simulink model "Envloads"  (R2021a)
settings: Solver=VariableStepAuto  StartTime=0.0  StopTime=100  RelTol=1e-3
undefined symbols (not defined in the file): alpha, C_phi, C_psi, C_tetha, Current_dir, Current_vel, Cx, Cy, mu, Umean, wind_dir_mean
libraries: mssSimulink x5, simulink x2
settings Model: Creator=premr  LastModifiedBy=premr

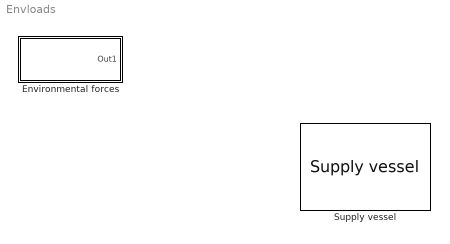
== system Envloads ==
  Environmental forces : Subsystem
  Supply vessel : mssSimulink/Marine craft models/Supply vessel  D=[5.0242e4 0 0; 0 2.7229e5 -4.3933e6; 0 -4.3933e6 4.1894e8]  Minv=inv( [5.3122e6 0 0; 0 8.2831e6 0; 0 0 3.7454e9] )

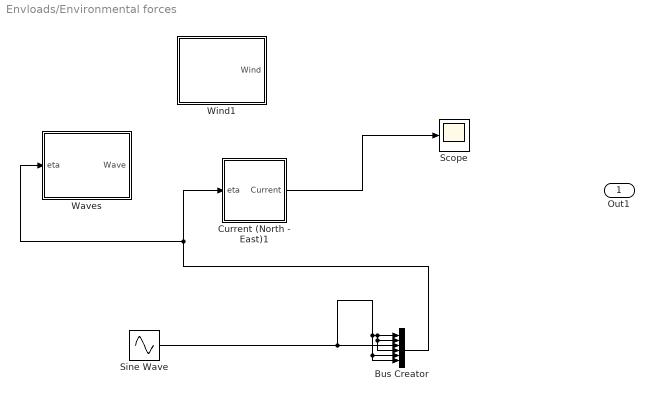
== system Envloads/Environmental forces ==
  Bus Creator : BusCreator  Inputs=6
  Current (North - East)1 : Subsystem
  Scope : Scope
  Sine Wave : Sin  Frequency=1/30  SampleTime=0
  Waves : Subsystem
  Wind1 : Subsystem
  Out1 : Outport
  wires:
  Sine Wave/1 -> Bus Creator/6, Bus Creator/5, Bus Creator/4, Bus Creator/2, Bus Creator/1, Bus Creator/3
  Bus Creator/1 -> Waves/1(eta), Current (North - East)1/1(eta)
  Current (North - East)1/1(Current) -> Scope/1

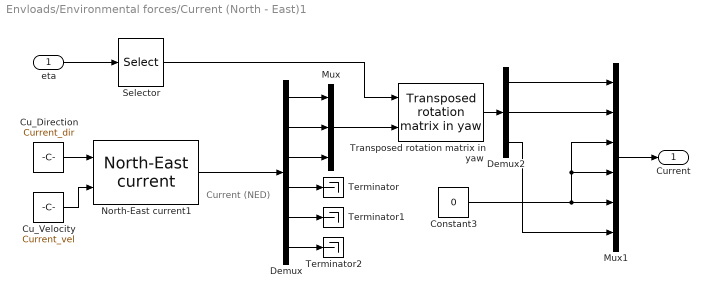
== system Envloads/Environmental forces/Current (North - East)1 ==
  note: Current (NED)
  eta : Inport
  Constant3 : Constant  Value=0
  Cu_Direction : Constant  Value=Current_dir
  Cu_Velocity : Constant  Value=Current_vel
  Demux : Demux  Outputs=6
  Demux2 : Demux  Outputs=3
  Mux : Mux  Inputs=3
  Mux1 : Mux  Inputs=6
  North-East current1 : mssSimulink/Environment/Current/North-East current  SystemSampleTime=-1  VariantActivationTime=update diagram  Latency=0  AutoFrameSizeCalculation=off
  Selector : Selector  InputPortWidth=6  IndexOptions=Index vector (dialog)  Indices=[6]  OutputSizes=1
  Terminator : Terminator
  Terminator1 : Terminator
  Terminator2 : Terminator
  Transposed rotation matrix in yaw : mssSimulink/Modelling/Kinematics/Transposed rotation  matrix in yaw
  Current : Outport  VectorParamsAs1DForOutWhenUnconnected=off
  wires:
  Constant3/1 -> Mux1/5, Mux1/4, Mux1/3
  Demux/6 -> Terminator2/1
  North-East current1/1 -> Demux/1
  Demux2/3 -> Mux1/6
  Demux/4 -> Terminator/1
  Demux/5 -> Terminator1/1
  Selector/1 -> Transposed rotation matrix in yaw/1
  Demux/3 -> Mux/3
  Mux/1 -> Transposed rotation matrix in yaw/2
  Demux/1 -> Mux/1
  Cu_Velocity/1 -> North-East current1/2
  Demux/2 -> Mux/2
  Mux1/1 -> Current/1
  Demux2/2 -> Mux1/2
  Transposed rotation matrix in yaw/1 -> Demux2/1
  eta/1 -> Selector/1
  Cu_Direction/1 -> North-East current1/1
  Demux2/1 -> Mux1/1

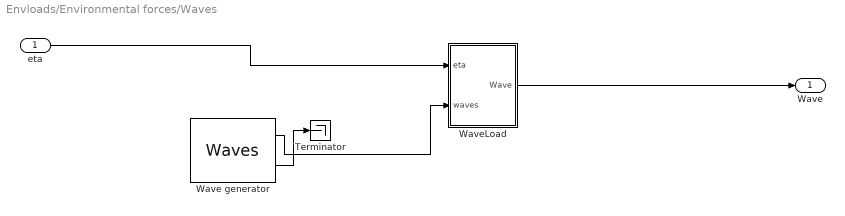
== system Envloads/Environmental forces/Waves ==
  eta : Inport
  Terminator : Terminator
  Wave generator : mssSimulink/Environment/Waves/Waves  spectrum_type=ITTC  disp_flag=on  plot_spectrum=off  plot_realization=off  hs=0.8  omega_peak=0  psi_mean=0  gamma=-1  spread=2  depth=inf  nfreq=20  ndir=10  energylim=0.005  freq_cutoff=3  dir_cutoff=0  rand_seed=123  rand_freq=on  rand_dir=on  Zeta_a=0  Omega=0  Phase=0  Wavenum=0  Psi=0
  WaveLoad : Subsystem  mask{waveforces=on}
      mask prompts: waveforces "Waveforces enabled"
  Wave : Outport  VectorParamsAs1DForOutWhenUnconnected=off
  wires:
  Wave generator/1 -> WaveLoad/2(waves)
  Wave generator/2 -> Terminator/1
  eta/1 -> WaveLoad/1(eta)
  WaveLoad/1(Wave) -> Wave/1

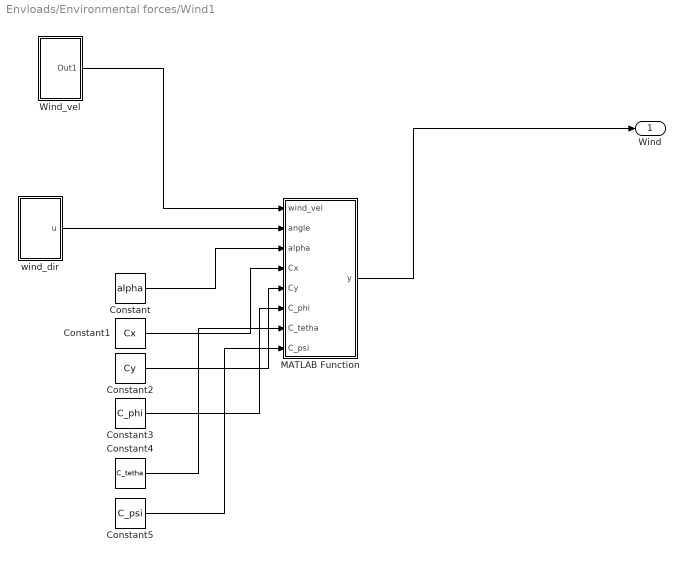
== system Envloads/Environmental forces/Wind1 ==
  Constant : Constant  Value=alpha
  Constant1 : Constant  Value=Cx
  Constant2 : Constant  Value=Cy
  Constant3 : Constant  Value=C_phi
  Constant4 : Constant  Value=C_tetha
  Constant5 : Constant  Value=C_psi
  MATLAB Function : MATLAB Function  TreatAsAtomicUnit=on
  Wind_vel : Subsystem
  wind_dir : Subsystem
  Wind : Outport  VectorParamsAs1DForOutWhenUnconnected=off
  wires:
  wind_dir/1(u) -> MATLAB Function/2(angle)
  Wind_vel/1(Out1) -> MATLAB Function/1(wind_vel)
  MATLAB Function/1(y) -> Wind/1
  Constant/1 -> MATLAB Function/3(alpha)
  Constant1/1 -> MATLAB Function/4(Cx)
  Constant2/1 -> MATLAB Function/5(Cy)
  Constant3/1 -> MATLAB Function/6(C_phi)
  Constant4/1 -> MATLAB Function/7(C_tetha)
  Constant5/1 -> MATLAB Function/8(C_psi)

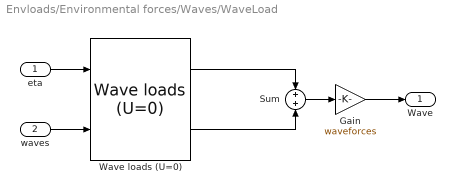
== system Envloads/Environmental forces/Waves/WaveLoad ==
  eta : Inport
  waves : Inport  Port=2
  Gain : Gain  Gain=waveforces
  Sum : Sum
  Wave loads (U=0) : mssSimulink/Hydrodynamics/Wave loads (U=0)  SystemSampleTime=-1  VariantActivationTime=update diagram  Latency=0  AutoFrameSizeCalculation=off
  Wave : Outport  VectorParamsAs1DForOutWhenUnconnected=off
  wires:
  eta/1 -> Wave loads (U=0)/1
  waves/1 -> Wave loads (U=0)/2
  Sum/1 -> Gain/1
  Wave loads (U=0)/1 -> Sum/1
  Wave loads (U=0)/2 -> Sum/2
  Gain/1 -> Wave/1

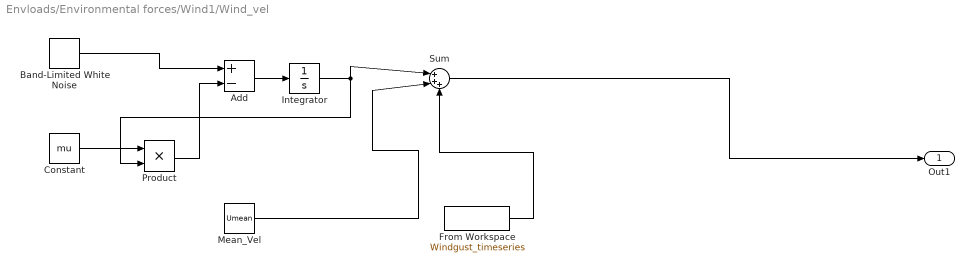
== system Envloads/Environmental forces/Wind1/Wind_vel ==
  Add : Sum  Inputs=+-
  Band-Limited White Noise : simulink/Sources/Band-Limited White Noise  Cov=[0.005]  Ts=0.1  seed=[23341]
  Constant : Constant  Value=mu
  From Workspace : FromWorkspace  VariableName=Windgust_timeseries  SampleTime=0.01
  Integrator : Integrator
  Mean_Vel : Constant  Value=Umean  SampleTime=1
  Product : Product
  Sum : Sum  Inputs=|+++
  Out1 : Outport
  wires:
  Integrator/1 -> Product/2, Sum/1
  Sum/1 -> Out1/1
  Mean_Vel/1 -> Sum/2
  Product/1 -> Add/2
  Add/1 -> Integrator/1
  From Workspace/1 -> Sum/3
  Band-Limited White Noise/1 -> Add/1
  Constant/1 -> Product/1

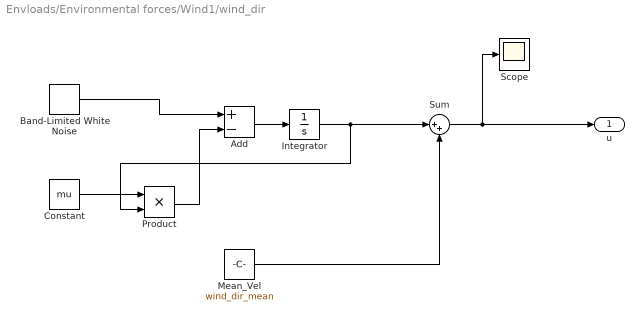
== system Envloads/Environmental forces/Wind1/wind_dir ==
  Add : Sum  Inputs=+-
  Band-Limited White Noise : simulink/Sources/Band-Limited White Noise  Cov=[0.005]  Ts=0.1  seed=[23341]
  Constant : Constant  Value=mu
  Integrator : Integrator
  Mean_Vel : Constant  Value=wind_dir_mean  SampleTime=1
  Product : Product
  Scope : Scope
  Sum : Sum  Inputs=|++
  u : Outport
  wires:
  Band-Limited White Noise/1 -> Add/1
  Add/1 -> Integrator/1
  Integrator/1 -> Product/2, Sum/1
  Sum/1 -> Scope/1, u/1
  Constant/1 -> Product/1
  Mean_Vel/1 -> Sum/2
  Product/1 -> Add/2

== matlab function Envloads/Environmental forces/Wind1/MATLAB Function ==
  data: wind_vel input; angle input; y output; alpha input; Cx input; Cy input; C_phi input; C_tetha input; C_psi input
function y = fcn(wind_vel, angle, alpha, Cx, Cy, C_phi, C_tetha, C_psi)
C1 = interp1(alpha,Cx,angle);  %if alpha is negative, add 360
C2 = interp1(alpha,Cy,angle);
C3 = 0;
C4 = interp1(alpha,C_phi,angle);
C5 = interp1(alpha,C_tetha,angle);
C6 = interp1(alpha,C_psi,angle);
y = transpose((wind_vel^2).*[C1 C2 C3 C4 C5 C6]);
